simulink model "psm_stromregelung"  (R2025a)
settings: Solver=VariableStepAuto  StartTime=0.0  StopTime=10.0  RelTol=1e-3
settings Model: Creator=moham  LastModifiedBy=moham

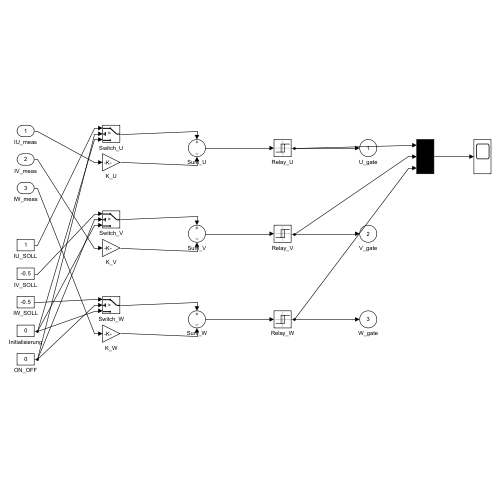
[thumbnail: Simulink's stored preview of the top-level diagram]
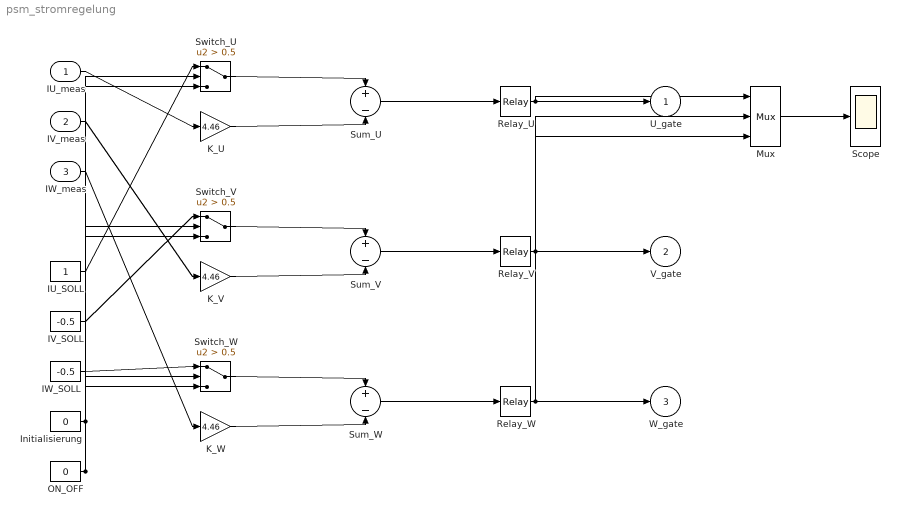
== system psm_stromregelung ==
  IU_meas : Inport
  IV_meas : Inport  Port=2
  IW_meas : Inport  Port=3
  IU_SOLL : Constant
  IV_SOLL : Constant  Value=-0.5
  IW_SOLL : Constant  Value=-0.5
  Initialisierung : Constant  Value=0
  K_U : Gain  Gain=4.46
  K_V : Gain  Gain=4.46
  K_W : Gain  Gain=4.46
  Mux : Mux  Inputs=3
  ON_OFF : Constant  Value=0
  Relay_U : Relay  OnSwitchValue=0.01  OffSwitchValue=-0.01
  Relay_V : Relay  OnSwitchValue=0.01  OffSwitchValue=-0.01
  Relay_W : Relay  OnSwitchValue=0.01  OffSwitchValue=-0.01
  Scope : Scope
  Sum_U : Sum  Inputs=+-
  Sum_V : Sum  Inputs=+-
  Sum_W : Sum  Inputs=+-
  Switch_U : Switch  Criteria=u2 > Threshold  Threshold=0.5  SaturateOnIntegerOverflow=off  InputSameDT=off
  Switch_V : Switch  Criteria=u2 > Threshold  Threshold=0.5  SaturateOnIntegerOverflow=off  InputSameDT=off
  Switch_W : Switch  Criteria=u2 > Threshold  Threshold=0.5  SaturateOnIntegerOverflow=off  InputSameDT=off
  U_gate : Outport
  V_gate : Outport  Port=2
  W_gate : Outport  Port=3
  wires:
  IU_SOLL/1 -> Switch_U/1
  ON_OFF/1 -> Switch_U/2, Switch_V/2, Switch_W/2
  Initialisierung/1 -> Switch_U/3, Switch_V/3, Switch_W/3
  IU_meas/1 -> K_U/1
  Switch_U/1 -> Sum_U/1
  K_U/1 -> Sum_U/2
  Sum_U/1 -> Relay_U/1
  Relay_U/1 -> U_gate/1, Mux/1
  IV_SOLL/1 -> Switch_V/1
  IV_meas/1 -> K_V/1
  Switch_V/1 -> Sum_V/1
  K_V/1 -> Sum_V/2
  Sum_V/1 -> Relay_V/1
  Relay_V/1 -> V_gate/1, Mux/2
  IW_SOLL/1 -> Switch_W/1
  IW_meas/1 -> K_W/1
  Switch_W/1 -> Sum_W/1
  K_W/1 -> Sum_W/2
  Sum_W/1 -> Relay_W/1
  Relay_W/1 -> W_gate/1, Mux/3
  Mux/1 -> Scope/1
